simulink model "InsulinPumpModelV7_ParFor"  (R2016b)
settings: Solver=ode23t  StartTime=0.0  StopTime=12  MaxStep=0.001  RelTol=1e-5  EnableMultiTasking=on
undefined symbols (not defined in the file): const, const_Occl_Pct, DeliveryType, DiscIntNeverNeededParam, MagB, PauseTime, StrokeTimeB
libraries: fl_lib x79, nesl_utility x35, sldvlib x14, sh_lib x9, sdl_lib x7, simulink x2, elec_lib x1, simulink_extras x1
(part 2 of 2)

== system InsulinPumpModelV7_ParFor/Plant/Reservoir2/TransSensor ==
  Ideal Translational Motion Sensor : fl_lib/Mechanical/Mechanical Sensors/Ideal Translational Motion Sensor  offset=0 m
  Mechanical Translational Reference1 : fl_lib/Mechanical/Translational Elements/Mechanical Translational Reference
  PS-Simulink Converter3 : nesl_utility/PS-Simulink Converter  PhysicalDomain=network_engine_domain  SubClassName=ps_output  LeftPortType=input  RightPortType=output  PseudoPeriodic=off  Frequencies=[]  Unit=mm/min  AffineConversion=off
  PS-Simulink Converter4 : nesl_utility/PS-Simulink Converter  PhysicalDomain=network_engine_domain  SubClassName=ps_output  LeftPortType=input  RightPortType=output  PseudoPeriodic=off  Frequencies=[]  Unit=mm  AffineConversion=off
  Scope : Scope
  Scope1 : Scope
  Terminator : Terminator
  Terminator1 : Terminator
  Conn1 : PMIOPort  Port=1  Side=Left
  P : PMIOPort  Port=2  Side=Right
  wires:
  PS-Simulink Converter3/1 -> Terminator/1, Scope/1  "Piston_V"
  PS-Simulink Converter4/1 -> Terminator1/1, Scope1/1  "Piston_P"
  connections:
  Mechanical Translational Reference1/LConn1 -- Ideal Translational Motion Sensor/RConn1
  PS-Simulink Converter3/LConn1 -- Ideal Translational Motion Sensor/RConn2
  PS-Simulink Converter4/LConn1 -- P/RConn1 -- Ideal Translational Motion Sensor/RConn3
  Conn1/RConn1 -- Ideal Translational Motion Sensor/LConn1

== system InsulinPumpModelV7_ParFor/Plant/Reservoir3/P Sensor ==
  Hydraulic Pressure Sensor : fl_lib/Hydraulic/Hydraulic Sensors/Hydraulic Pressure Sensor
  Hydraulic Reference : fl_lib/Hydraulic/Hydraulic Elements/Hydraulic Reference
  PS-Simulink Converter : nesl_utility/PS-Simulink Converter  PhysicalDomain=network_engine_domain  SubClassName=ps_output  LeftPortType=input  RightPortType=output  PseudoPeriodic=off  Frequencies=[]  Unit=1  AffineConversion=off
  Scope1 : Scope
  A : PMIOPort  Port=1  Side=Left
  wires:
  PS-Simulink Converter/1 -> Scope1/1  "Press1"
  connections:
  A/RConn1 -- Hydraulic Pressure Sensor/LConn1
  Hydraulic Pressure Sensor/RConn2 -- PS-Simulink Converter/LConn1
  Hydraulic Pressure Sensor/RConn1 -- Hydraulic Reference/LConn1

== system InsulinPumpModelV7_ParFor/Plant/Reservoir3/TransSensor ==
  Ideal Translational Motion Sensor : fl_lib/Mechanical/Mechanical Sensors/Ideal Translational Motion Sensor  offset=0 m
  Mechanical Translational Reference1 : fl_lib/Mechanical/Translational Elements/Mechanical Translational Reference
  PS-Simulink Converter3 : nesl_utility/PS-Simulink Converter  PhysicalDomain=network_engine_domain  SubClassName=ps_output  LeftPortType=input  RightPortType=output  PseudoPeriodic=off  Frequencies=[]  Unit=mm/min  AffineConversion=off
  PS-Simulink Converter4 : nesl_utility/PS-Simulink Converter  PhysicalDomain=network_engine_domain  SubClassName=ps_output  LeftPortType=input  RightPortType=output  PseudoPeriodic=off  Frequencies=[]  Unit=mm  AffineConversion=off
  Scope : Scope
  Scope1 : Scope
  Terminator : Terminator
  Terminator1 : Terminator
  Conn1 : PMIOPort  Port=1  Side=Left
  P : PMIOPort  Port=2  Side=Right
  wires:
  PS-Simulink Converter3/1 -> Terminator/1, Scope/1  "Piston_V"
  PS-Simulink Converter4/1 -> Terminator1/1, Scope1/1  "Piston_P"
  connections:
  Mechanical Translational Reference1/LConn1 -- Ideal Translational Motion Sensor/RConn1
  PS-Simulink Converter3/LConn1 -- Ideal Translational Motion Sensor/RConn2
  PS-Simulink Converter4/LConn1 -- P/RConn1 -- Ideal Translational Motion Sensor/RConn3
  Conn1/RConn1 -- Ideal Translational Motion Sensor/LConn1

== system InsulinPumpModelV7_ParFor/Plant/Slide1/Force Sensor ==
  Ideal Force Sensor1 : fl_lib/Mechanical/Mechanical Sensors/Ideal Force Sensor
  PS-Simulink Converter15 : nesl_utility/PS-Simulink Converter  PhysicalDomain=network_engine_domain  SubClassName=ps_output  LeftPortType=input  RightPortType=output  PseudoPeriodic=off  Frequencies=[]  Unit=N  AffineConversion=off
  Rate Transition4 : RateTransition  OutPortSampleTime=0.01
  Scope2 : Scope
  Terminator : Terminator
  C : PMIOPort  Port=1  Side=Right
  R : PMIOPort  Port=2  Side=Left
  wires:
  PS-Simulink Converter15/1 -> Rate Transition4/1, Terminator/1  "Slide_Force"
  Rate Transition4/1 -> Scope2/1
  connections:
  Ideal Force Sensor1/LConn1 -- R/RConn1
  PS-Simulink Converter15/LConn1 -- Ideal Force Sensor1/RConn2
  C/RConn1 -- Ideal Force Sensor1/RConn1

== system InsulinPumpModelV7_ParFor/Plant/Slide2/Force Sensor ==
  Ideal Force Sensor1 : fl_lib/Mechanical/Mechanical Sensors/Ideal Force Sensor
  PS-Simulink Converter15 : nesl_utility/PS-Simulink Converter  PhysicalDomain=network_engine_domain  SubClassName=ps_output  LeftPortType=input  RightPortType=output  PseudoPeriodic=off  Frequencies=[]  Unit=N  AffineConversion=off
  Rate Transition4 : RateTransition  OutPortSampleTime=0.01
  Scope2 : Scope
  Terminator : Terminator
  C : PMIOPort  Port=1  Side=Right
  R : PMIOPort  Port=2  Side=Left
  wires:
  Rate Transition4/1 -> Scope2/1
  PS-Simulink Converter15/1 -> Terminator/1, Rate Transition4/1  "Slide_Force"
  connections:
  C/RConn1 -- Ideal Force Sensor1/RConn1
  PS-Simulink Converter15/LConn1 -- Ideal Force Sensor1/RConn2
  Ideal Force Sensor1/LConn1 -- R/RConn1

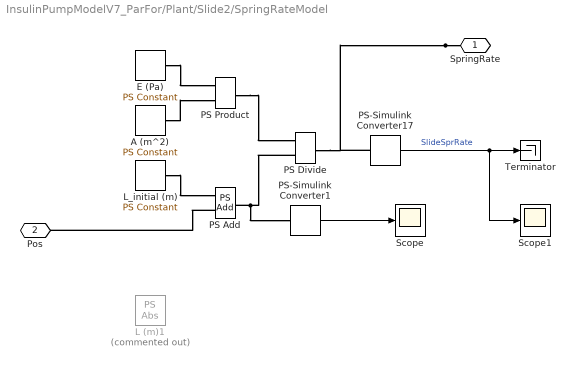
== system InsulinPumpModelV7_ParFor/Plant/Slide2/SpringRateModel ==
  A (m^2) : fl_lib/Physical Signals/Sources/PS Constant  constant=A
  E (Pa) : fl_lib/Physical Signals/Sources/PS Constant  constant=E
  L (m)1 : fl_lib/Physical Signals/Nonlinear Operators/PS Abs  Commented=on
  L_initial (m) : fl_lib/Physical Signals/Sources/PS Constant  constant=InitL
  PS Add : fl_lib/Physical Signals/Functions/PS Add
  PS Divide : fl_lib/Physical Signals/Functions/PS Divide
  PS Product : fl_lib/Physical Signals/Functions/PS Product
  PS-Simulink Converter1 : nesl_utility/PS-Simulink Converter  PhysicalDomain=network_engine_domain  SubClassName=ps_output  LeftPortType=input  RightPortType=output  PseudoPeriodic=off  Frequencies=[]  Unit=N/m  AffineConversion=off
  PS-Simulink Converter17 : nesl_utility/PS-Simulink Converter  PhysicalDomain=network_engine_domain  SubClassName=ps_output  LeftPortType=input  RightPortType=output  PseudoPeriodic=off  Frequencies=[]  Unit=N/m  AffineConversion=off
  Scope : Scope
  Scope1 : Scope
  Terminator : Terminator
  SpringRate : PMIOPort  Port=1  Side=Right
  Pos : PMIOPort  Port=2  Side=Left
  wires:
  PS-Simulink Converter1/1 -> Scope/1
  PS-Simulink Converter17/1 -> Terminator/1, Scope1/1  "SlideSprRate"
  connections:
  PS Add/LConn2 -- Pos/RConn1
  PS Add/RConn1 -- PS-Simulink Converter1/LConn1 -- PS Divide/LConn2
  L_initial (m)/RConn1 -- PS Add/LConn1
  SpringRate/RConn1 -- PS-Simulink Converter17/LConn1 -- PS Divide/RConn1
  PS Product/RConn1 -- PS Divide/LConn1
  A (m^2)/RConn1 -- PS Product/LConn2
  E (Pa)/RConn1 -- PS Product/LConn1

== system InsulinPumpModelV7_ParFor/Plant/Slide2/TransSensor ==
  Ideal Translational Motion Sensor : fl_lib/Mechanical/Mechanical Sensors/Ideal Translational Motion Sensor  offset=0 m
  Mechanical Translational Reference1 : fl_lib/Mechanical/Translational Elements/Mechanical Translational Reference
  PS-Simulink Converter3 : nesl_utility/PS-Simulink Converter  PhysicalDomain=network_engine_domain  SubClassName=ps_output  LeftPortType=input  RightPortType=output  PseudoPeriodic=off  Frequencies=[]  Unit=mm/s  AffineConversion=off
  PS-Simulink Converter4 : nesl_utility/PS-Simulink Converter  PhysicalDomain=network_engine_domain  SubClassName=ps_output  LeftPortType=input  RightPortType=output  PseudoPeriodic=off  Frequencies=[]  Unit=mm  AffineConversion=off
  Terminator : Terminator
  Terminator1 : Terminator
  Conn1 : PMIOPort  Port=1  Side=Left
  P : PMIOPort  Port=2  Side=Right
  wires:
  PS-Simulink Converter3/1 -> Terminator/1  "Slide_V"
  PS-Simulink Converter4/1 -> Terminator1/1  "Slide_P"
  connections:
  Mechanical Translational Reference1/LConn1 -- Ideal Translational Motion Sensor/RConn1
  PS-Simulink Converter3/LConn1 -- Ideal Translational Motion Sensor/RConn2
  PS-Simulink Converter4/LConn1 -- P/RConn1 -- Ideal Translational Motion Sensor/RConn3
  Conn1/RConn1 -- Ideal Translational Motion Sensor/LConn1

== system InsulinPumpModelV7_ParFor/Plant/Slide3/Force Sensor ==
  Ideal Force Sensor1 : fl_lib/Mechanical/Mechanical Sensors/Ideal Force Sensor
  PS-Simulink Converter15 : nesl_utility/PS-Simulink Converter  PhysicalDomain=network_engine_domain  SubClassName=ps_output  LeftPortType=input  RightPortType=output  PseudoPeriodic=off  Frequencies=[]  Unit=N  AffineConversion=off
  Rate Transition4 : RateTransition  OutPortSampleTime=0.01
  Scope2 : Scope
  Terminator : Terminator
  C : PMIOPort  Port=1  Side=Right
  R : PMIOPort  Port=2  Side=Left
  wires:
  Rate Transition4/1 -> Scope2/1
  PS-Simulink Converter15/1 -> Terminator/1, Rate Transition4/1  "Slide_Force"
  connections:
  C/RConn1 -- Ideal Force Sensor1/RConn1
  PS-Simulink Converter15/LConn1 -- Ideal Force Sensor1/RConn2
  Ideal Force Sensor1/LConn1 -- R/RConn1

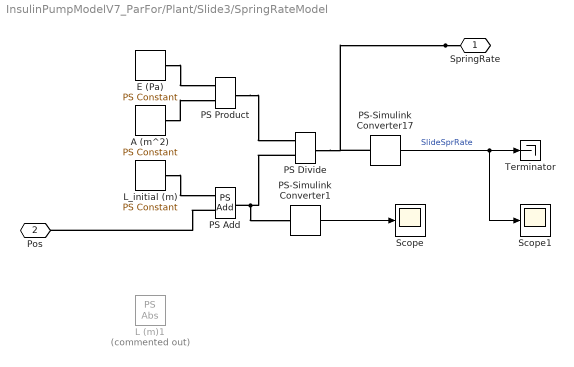
== system InsulinPumpModelV7_ParFor/Plant/Slide3/SpringRateModel ==
  A (m^2) : fl_lib/Physical Signals/Sources/PS Constant  constant=A
  E (Pa) : fl_lib/Physical Signals/Sources/PS Constant  constant=E
  L (m)1 : fl_lib/Physical Signals/Nonlinear Operators/PS Abs  Commented=on
  L_initial (m) : fl_lib/Physical Signals/Sources/PS Constant  constant=InitL
  PS Add : fl_lib/Physical Signals/Functions/PS Add
  PS Divide : fl_lib/Physical Signals/Functions/PS Divide
  PS Product : fl_lib/Physical Signals/Functions/PS Product
  PS-Simulink Converter1 : nesl_utility/PS-Simulink Converter  PhysicalDomain=network_engine_domain  SubClassName=ps_output  LeftPortType=input  RightPortType=output  PseudoPeriodic=off  Frequencies=[]  Unit=N/m  AffineConversion=off
  PS-Simulink Converter17 : nesl_utility/PS-Simulink Converter  PhysicalDomain=network_engine_domain  SubClassName=ps_output  LeftPortType=input  RightPortType=output  PseudoPeriodic=off  Frequencies=[]  Unit=N/m  AffineConversion=off
  Scope : Scope
  Scope1 : Scope
  Terminator : Terminator
  SpringRate : PMIOPort  Port=1  Side=Right
  Pos : PMIOPort  Port=2  Side=Left
  wires:
  PS-Simulink Converter1/1 -> Scope/1
  PS-Simulink Converter17/1 -> Terminator/1, Scope1/1  "SlideSprRate"
  connections:
  PS Add/LConn2 -- Pos/RConn1
  PS Add/RConn1 -- PS-Simulink Converter1/LConn1 -- PS Divide/LConn2
  L_initial (m)/RConn1 -- PS Add/LConn1
  SpringRate/RConn1 -- PS-Simulink Converter17/LConn1 -- PS Divide/RConn1
  PS Product/RConn1 -- PS Divide/LConn1
  A (m^2)/RConn1 -- PS Product/LConn2
  E (Pa)/RConn1 -- PS Product/LConn1

== system InsulinPumpModelV7_ParFor/Plant/Slide3/TransSensor ==
  Ideal Translational Motion Sensor : fl_lib/Mechanical/Mechanical Sensors/Ideal Translational Motion Sensor  offset=0 m
  Mechanical Translational Reference1 : fl_lib/Mechanical/Translational Elements/Mechanical Translational Reference
  PS-Simulink Converter3 : nesl_utility/PS-Simulink Converter  PhysicalDomain=network_engine_domain  SubClassName=ps_output  LeftPortType=input  RightPortType=output  PseudoPeriodic=off  Frequencies=[]  Unit=mm/s  AffineConversion=off
  PS-Simulink Converter4 : nesl_utility/PS-Simulink Converter  PhysicalDomain=network_engine_domain  SubClassName=ps_output  LeftPortType=input  RightPortType=output  PseudoPeriodic=off  Frequencies=[]  Unit=mm  AffineConversion=off
  Terminator : Terminator
  Terminator1 : Terminator
  Conn1 : PMIOPort  Port=1  Side=Left
  P : PMIOPort  Port=2  Side=Right
  wires:
  PS-Simulink Converter3/1 -> Terminator/1  "Slide_V"
  PS-Simulink Converter4/1 -> Terminator1/1  "Slide_P"
  connections:
  Mechanical Translational Reference1/LConn1 -- Ideal Translational Motion Sensor/RConn1
  PS-Simulink Converter3/LConn1 -- Ideal Translational Motion Sensor/RConn2
  PS-Simulink Converter4/LConn1 -- P/RConn1 -- Ideal Translational Motion Sensor/RConn3
  Conn1/RConn1 -- Ideal Translational Motion Sensor/LConn1

== system InsulinPumpModelV7_ParFor/Subsystem/SpeedController/FeedbackController ==
  RefASpd : Inport  OutMin=-6000  OutMax=6000
  ASpd : Inport  Port=2  OutMin=-6000  OutMax=6000
  1-D Lookup Table : Lookup_n-D  NumberOfTableDimensions=1  BreakpointsForDimension1=[0 12.8 33.8 450]  Table=[1 1 1 1]*5e-4  InternalRulePriority=Speed  RndMeth=Simplest  InputSameDT=on
  1-D Lookup Table1 : Lookup_n-D  NumberOfTableDimensions=1  BreakpointsForDimension1=[0 12.8 33.8 450]  Table=[1 1 1 1]*5e-4  InternalRulePriority=Speed  RndMeth=Simplest  InputSameDT=on
  Add : Sum  Inputs=+-
  PID Controller : simulink/Continuous/PID Controller  Controller=PI  TimeDomain=Discrete-time  SampleTime=0.001  IntegratorMethod=Forward Euler  FilterMethod=Forward Euler  Form=Parallel  UseFilter=on  ControllerParametersSource=external  P=2e-3  I=2e-3  D=0  N=100  InitialConditionSource=internal  InitialConditionForIntegrator=0  InitialConditionForFilter=0  ExternalReset=none  LimitOutput=off  UpperSaturationLimit=1  LowerSaturationLimit=1  LinearizeAsGain=on  AntiWindupMode=clamping  Kb=1  TrackingMode=off  Kt=1  PParamMin=[]  PParamMax=[]  IParamMin=[]  IParamMax=[]  DParamMin=[]  DParamMax=[]  NParamMin=[]  NParamMax=[]  KbParamMin=[]  KbParamMax=[]  KtParamMin=[]  KtParamMax=[]  POutMin=[]  POutMax=[]  IOutMin=[]  IOutMax=[]  DOutMin=[]  DOutMax=[]  NOutMin=[]  NOutMax=[]  KbOutMin=[]  KbOutMax=[]  KtOutMin=[]  KtOutMax=[]  IntegratorOutMin=[]  IntegratorOutMax=[]  FilterOutMin=[]  FilterOutMax=[]  SumOutMin=[]  SumOutMax=[]  SumI1OutMin=[]  SumI1OutMax=[]  SumI2OutMin=[]  SumI2OutMax=[]  SumI3OutMin=[]  SumI3OutMax=[]  SumDOutMin=[]  SumDOutMax=[]  SaturationOutMin=[]  SaturationOutMax=[]  IntegratorContinuousStateAttributes=''  IntegratorStateMustResolveToSignalObject=off  IntegratorRTWStateStorageClass=Auto  FilterContinuousStateAttributes=''  FilterStateMustResolveToSignalObject=off  FilterRTWStateStorageClass=Auto  DifferentiatorICPrevScaledInput=0  DifferentiatorOutMin=[]  DifferentiatorOutMax=[]
  Volt : Outport  OutMin=-10  OutMax=10
  wires:
  ASpd/1 -> Add/2
  Add/1 -> 1-D Lookup Table1/1, 1-D Lookup Table/1, PID Controller/1
  PID Controller/1 -> Volt/1
  1-D Lookup Table/1 -> PID Controller/2
  1-D Lookup Table1/1 -> PID Controller/3
  RefASpd/1 -> Add/1

== system InsulinPumpModelV7_ParFor/Subsystem/Units_Conversion/BasalMap2Spd ==
  unit/hr : Inport
  1/CrossArea_Output(mm/min) : Gain  Gain=1/const.Resvor.Area
  Gain : Gain  Gain=1/60
  Gain3 : Gain  Gain=15
  Gear_Input(rev/min) : Gain  Gain=const.DriveSys.GearRatio
  Rev/inch_Output(rev/min) : Gain  Gain=1/const.DriveSys.ScrewLead
  mm2inch_Output(inch/min) : Gain  Gain=1/25.4
  rev/min : Outport
  wires:
  Gain/1 -> Gain3/1
  Gain3/1 -> 1/CrossArea_Output(mm/min)/1  "mm^3/min"
  mm2inch_Output(inch/min)/1 -> Rev/inch_Output(rev/min)/1
  unit/hr/1 -> Gain/1
  1/CrossArea_Output(mm/min)/1 -> mm2inch_Output(inch/min)/1
  Rev/inch_Output(rev/min)/1 -> Gear_Input(rev/min)/1
  Gear_Input(rev/min)/1 -> rev/min/1

== system InsulinPumpModelV7_ParFor/Subsystem/Units_Conversion/BolusMap2Spd ==
  unit/s : Inport
  1/CrossArea_Output(mm/min) : Gain  Gain=1/const.Resvor.Area
  Gain : Gain  Gain=60
  Gain3 : Gain  Gain=15
  Gear_Input(rev/min) : Gain  Gain=const.DriveSys.GearRatio
  Rev/inch_Output(rev/min) : Gain  Gain=1/const.DriveSys.ScrewLead
  mm2inch_Output(inch/min) : Gain  Gain=1/25.4
  rev/min : Outport
  wires:
  Rev/inch_Output(rev/min)/1 -> Gear_Input(rev/min)/1
  1/CrossArea_Output(mm/min)/1 -> mm2inch_Output(inch/min)/1
  unit/s/1 -> Gain/1
  mm2inch_Output(inch/min)/1 -> Rev/inch_Output(rev/min)/1
  Gain3/1 -> 1/CrossArea_Output(mm/min)/1  "mm^3/min"
  Gain/1 -> Gain3/1
  Gear_Input(rev/min)/1 -> rev/min/1

== stateflow chart InsulinPumpModelV7_ParFor/Subsystem/BolusChart ==
  state Off
  state NormalBolusMode
    state UnitRemainLow
    state NumCycFinished
    state Deliver
      entry: StrokeMag = MagB/StrokeTimeB;
    state Active
      entry: i = int8(0);
    state Pause
      entry: StrokeMag = single(0);
    state Inactive
      entry:StrokeMag = single(0);
    UnitRemainLow -> (junction 108)
    (junction 108) -> NormalBolusMode.Inactive
    (junction 27) -> UnitRemainLow [order 2] : [UnitRemain<LowLim+MagB]
    NumCycFinished -> (junction 41)
    (junction 41) -> NormalBolusMode.Inactive
    (junction 29) -> NumCycFinished [order 1] : [i>=NumCyc]
    (default) -> NormalBolusMode.Inactive
    Deliver -> (junction 104) : after(StrokeTimeB,sec)
    (junction 104) -> (junction 29) : {i = i + 1;}
    (junction 29) -> (junction 27) [order 2]
    (junction 27) -> Pause [order 1] : [UnitRemain>LowLim+MagB]
    NormalBolusMode.Inactive -> (junction 100) : [UnitRemain>LowLim+MagB]
    (junction 100) -> NormalBolusMode.Active : [DeliveryActive == true]
    NormalBolusMode.Active -> Deliver [order 1] : [i<NumCyc]
    Pause -> Deliver : after(PauseTime,sec)
    NormalBolusMode.Active -> NormalBolusMode.Inactive [order 2] : [UnitRemain<LowLim+MagB]
  state Armed
  state QuickBolusMode
    state Deliver1
      entry: StrokeMag = MagQB (1)/StrokeTimeQB(1);
    state Pause1
      entry: StrokeMag = single(0);
    state Inactive
      entry:StrokeMag = single(0);
    state Active
      entry: i = int8(0);
    state Deliver2
      entry: StrokeMag = MagQB(2)/StrokeTimeQB(2);
    state Pause2
      entry: StrokeMag = single(0);
    state Deliver3
      entry: StrokeMag = MagQB(3)/StrokeTimeQB(3);
    state Pause3
      entry: StrokeMag = single(0);
    state Deliver4
      entry: StrokeMag = MagQB(4)/StrokeTimeQB(4);
    state Pause4
      entry: StrokeMag = single(0);
    (junction 92) -> (junction 90)
    (junction 90) -> Deliver1
    Pause4 -> (junction 92) : after(PauseTime,sec)
    (default) -> QuickBolusMode.Inactive
    QuickBolusMode.Inactive -> (junction 119) : [UnitRemain>LowLim+sum(MagQB)]
    (junction 119) -> QuickBolusMode.Active : [DeliveryActive == true]
    QuickBolusMode.Active -> Deliver1
    Deliver1 -> Pause1 : after(StrokeTimeQB(1),sec)
    Pause1 -> Deliver2 : after(PauseTime,sec)
    (junction 116) -> QuickBolusMode.Inactive
    (junction 85) -> QuickBolusMode.Inactive
    Deliver2 -> Pause2 : after(StrokeTimeQB(2),sec)
    Pause2 -> Deliver3 : after(PauseTime,sec)
    Deliver3 -> Pause3 : after(StrokeTimeQB(3),sec)
    Pause3 -> Deliver4 : after(PauseTime,sec)
    Deliver4 -> (junction 78) : after(StrokeTimeQB(4),sec)
    (junction 78) -> (junction 77) : {i=i+1;}
    (junction 77) -> (junction 112) [order 1] : [i<NumCyc]
    (junction 112) -> Pause4 [order 1] : [UnitRemain>LowLim+sum(MagQB)]
    (junction 77) -> (junction 81) [order 2] : [i>=NumCyc]
    (junction 112) -> (junction 114) [order 2] : [UnitRemain<LowLim+sum(MagQB)]
    (junction 81) -> (junction 85)
    (junction 114) -> (junction 116)
  (default) -> Off
  Off -> Armed : [PowerOn ==true]
  Armed -> Off [order 1] : [PowerOn==false]
  Armed -> NormalBolusMode [order 2] : [DeliveryType ==1]
  NormalBolusMode -> Armed : [DeliveryType~=1]
  Armed -> QuickBolusMode [order 3] : [DeliveryType==2]
  QuickBolusMode -> Armed : [DeliveryType~=2]
  data: PowerOn input boolean [0..1]; DeliveryType input int8 [0..2]; NumCyc input int8 [0..100]; DeliveryActive input boolean [0..1]; MagB input single [0..3]; StrokeMag output [0..15]; i local int8; StrokeTimeB input single [0.2..5]; MagQB input single [0..3]; StrokeTimeQB input single [0.2..5]; PauseTime input single [0..100]; LowLim input single [0..100]; UnitRemain input single [0..201]

== stateflow chart InsulinPumpModelV7_ParFor/Subsystem/BasalChart ==
  state Off
  state On
  state BasalOff
    entry: BasalRate = single(0);
  state BasalOn
    entry:BasalRate = BasalSet;
  (default) -> Off
  Off -> On : [PowerOn ==true]
  On -> Off [order 1] : [PowerOn==false]
  On -> BasalOff [order 2] : [UnitRemain>LowLim]
  BasalOff -> BasalOn [order 2] : [BasalActive==true]
  BasalOn -> BasalOff [order 1] : [BasalActive==false]
  BasalOn -> BasalOff [order 2] : [UnitRemain<LowLim]
  BasalOff -> On [order 1] : [UnitRemain<LowLim]
  data: PowerOn input boolean [0..1]; BasalActive input boolean [0..1]; BasalSet input single [0..2]; LowLim input single [0..100]; UnitRemain input single [0..201]; BasalRate output single [0..2]
